simulink library "Byte_Multiplexers_Lib"  (Simulink 8.7)
settings: Solver=ode45  StartTime=0.0  StopTime=10.0  RelTol=1e-3
libraries: commutil2 x34, Bit_Multiplexers_Lib x32, Byte_Multiplexers_Lib x1, Encoders_Lib x1
settings Model: Creator=uzivatel  LastModifiedBy=Jozko Mrkvicka

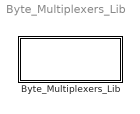
== system Byte_Multiplexers_Lib ==
  Byte_Multiplexers_Lib : Subsystem

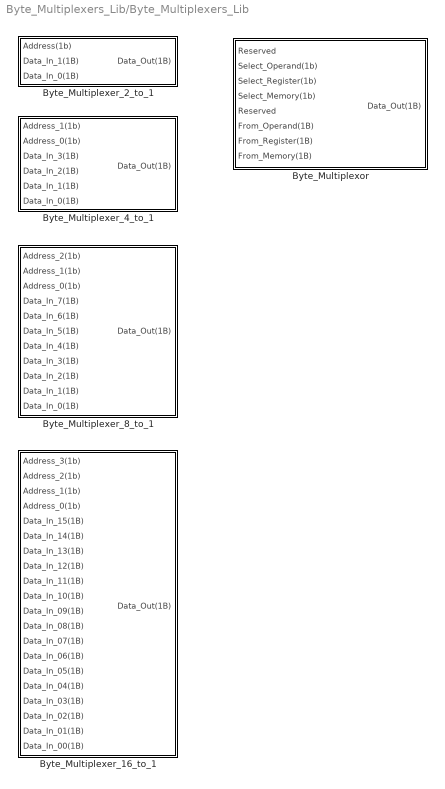
== system Byte_Multiplexers_Lib/Byte_Multiplexers_Lib ==
  Byte_Multiplexer_16_to_1 : Subsystem
  Byte_Multiplexer_2_to_1 : Subsystem
  Byte_Multiplexer_4_to_1 : Subsystem
  Byte_Multiplexer_8_to_1 : Subsystem
  Byte_Multiplexor : Subsystem

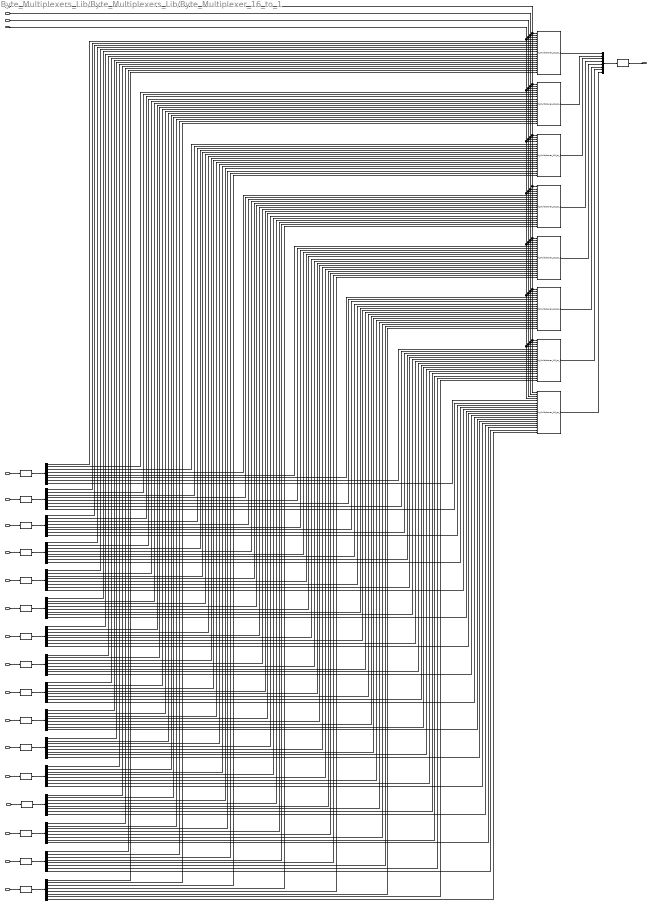
== system Byte_Multiplexers_Lib/Byte_Multiplexers_Lib/Byte_Multiplexer_16_to_1 ==
  Address_3(1b) : Inport
  Address_2(1b) : Inport  Port=2
  Address_1(1b) : Inport  Port=3
  Address_0(1b) : Inport  Port=4
  Data_In_15(1B) : Inport  Port=5
  Data_In_14(1B) : Inport  Port=6
  Data_In_13(1B) : Inport  Port=7
  Data_In_12(1B) : Inport  Port=8
  Data_In_11(1B) : Inport  Port=9
  Data_In_10(1B) : Inport  Port=10
  Data_In_09(1B) : Inport  Port=11
  Data_In_08(1B) : Inport  Port=12
  Data_In_07(1B) : Inport  Port=13
  Data_In_06(1B) : Inport  Port=14
  Data_In_05(1B) : Inport  Port=15
  Data_In_04(1B) : Inport  Port=16
  Data_In_03(1B) : Inport  Port=17
  Data_In_02(1B) : Inport  Port=18
  Data_In_01(1B) : Inport  Port=19
  Data_In_00(1B) : Inport  Port=20
  Bit to Integer Converter1 : commutil2/Bit to Integer Converter  nbits=8  bitOrder=MSB first  signedOutputValues=Unsigned  outDtype=uint8  outDtypeSigned=Inherit via internal rule
  Bit_Multiplexer_16_to_1(Bit_0) : Bit_Multiplexers_Lib/Bit_Multiplexers_Lib/Bit_Multiplexer_16_to_1
  Bit_Multiplexer_16_to_1(Bit_1) : Bit_Multiplexers_Lib/Bit_Multiplexers_Lib/Bit_Multiplexer_16_to_1
  Bit_Multiplexer_16_to_1(Bit_2) : Bit_Multiplexers_Lib/Bit_Multiplexers_Lib/Bit_Multiplexer_16_to_1
  Bit_Multiplexer_16_to_1(Bit_3) : Bit_Multiplexers_Lib/Bit_Multiplexers_Lib/Bit_Multiplexer_16_to_1
  Bit_Multiplexer_16_to_1(Bit_4) : Bit_Multiplexers_Lib/Bit_Multiplexers_Lib/Bit_Multiplexer_16_to_1
  Bit_Multiplexer_16_to_1(Bit_5) : Bit_Multiplexers_Lib/Bit_Multiplexers_Lib/Bit_Multiplexer_16_to_1
  Bit_Multiplexer_16_to_1(Bit_6) : Bit_Multiplexers_Lib/Bit_Multiplexers_Lib/Bit_Multiplexer_16_to_1
  Bit_Multiplexer_16_to_1(Bit_7) : Bit_Multiplexers_Lib/Bit_Multiplexers_Lib/Bit_Multiplexer_16_to_1
  Byte_{0..15} (16 alike) : Demux  Outputs=8
  Integer to Bit Converter{1..16} (16 alike) : commutil2/Integer to Bit Converter  nbits=8  signedInputValues=Unsigned  bitOrder=MSB first  outDtype=boolean
  Mux : Mux  Inputs=8
  Data_Out(1B) : Outport
  wires:
  Integer to Bit Converter7/1 -> Byte_15/1
  Data_In_15(1B)/1 -> Integer to Bit Converter7/1
  Mux/1 -> Bit to Integer Converter1/1
  Bit to Integer Converter1/1 -> Data_Out(1B)/1
  Address_0(1b)/1 -> Bit_Multiplexer_16_to_1(Bit_5)/4, Bit_Multiplexer_16_to_1(Bit_0)/4, Bit_Multiplexer_16_to_1(Bit_1)/4, Bit_Multiplexer_16_to_1(Bit_2)/4, Bit_Multiplexer_16_to_1(Bit_3)/4, Bit_Multiplexer_16_to_1(Bit_4)/4, Bit_Multiplexer_16_to_1(Bit_6)/4, Bit_Multiplexer_16_to_1(Bit_7)/4
  Address_1(1b)/1 -> Bit_Multiplexer_16_to_1(Bit_5)/3, Bit_Multiplexer_16_to_1(Bit_0)/3, Bit_Multiplexer_16_to_1(Bit_1)/3, Bit_Multiplexer_16_to_1(Bit_2)/3, Bit_Multiplexer_16_to_1(Bit_3)/3, Bit_Multiplexer_16_to_1(Bit_4)/3, Bit_Multiplexer_16_to_1(Bit_6)/3, Bit_Multiplexer_16_to_1(Bit_7)/3
  Address_2(1b)/1 -> Bit_Multiplexer_16_to_1(Bit_6)/2, Bit_Multiplexer_16_to_1(Bit_5)/2, Bit_Multiplexer_16_to_1(Bit_4)/2, Bit_Multiplexer_16_to_1(Bit_2)/2, Bit_Multiplexer_16_to_1(Bit_1)/2, Bit_Multiplexer_16_to_1(Bit_0)/2, Bit_Multiplexer_16_to_1(Bit_3)/2, Bit_Multiplexer_16_to_1(Bit_7)/2
  Address_3(1b)/1 -> Bit_Multiplexer_16_to_1(Bit_5)/1, Bit_Multiplexer_16_to_1(Bit_0)/1, Bit_Multiplexer_16_to_1(Bit_1)/1, Bit_Multiplexer_16_to_1(Bit_2)/1, Bit_Multiplexer_16_to_1(Bit_3)/1, Bit_Multiplexer_16_to_1(Bit_4)/1, Bit_Multiplexer_16_to_1(Bit_6)/1, Bit_Multiplexer_16_to_1(Bit_7)/1
  Bit_Multiplexer_16_to_1(Bit_4)/1 -> Mux/4
  Bit_Multiplexer_16_to_1(Bit_5)/1 -> Mux/3
  Bit_Multiplexer_16_to_1(Bit_6)/1 -> Mux/2
  Bit_Multiplexer_16_to_1(Bit_7)/1 -> Mux/1
  Bit_Multiplexer_16_to_1(Bit_3)/1 -> Mux/5
  Bit_Multiplexer_16_to_1(Bit_2)/1 -> Mux/6
  Bit_Multiplexer_16_to_1(Bit_1)/1 -> Mux/7
  Bit_Multiplexer_16_to_1(Bit_0)/1 -> Mux/8
  Integer to Bit Converter1/1 -> Byte_14/1
  Data_In_14(1B)/1 -> Integer to Bit Converter1/1
  Integer to Bit Converter2/1 -> Byte_13/1
  Data_In_13(1B)/1 -> Integer to Bit Converter2/1
  Integer to Bit Converter3/1 -> Byte_12/1
  Data_In_12(1B)/1 -> Integer to Bit Converter3/1
  Integer to Bit Converter4/1 -> Byte_11/1
  Data_In_11(1B)/1 -> Integer to Bit Converter4/1
  Integer to Bit Converter5/1 -> Byte_10/1
  Data_In_10(1B)/1 -> Integer to Bit Converter5/1
  Integer to Bit Converter6/1 -> Byte_9/1
  Data_In_09(1B)/1 -> Integer to Bit Converter6/1
  Integer to Bit Converter8/1 -> Byte_8/1
  Data_In_08(1B)/1 -> Integer to Bit Converter8/1
  Integer to Bit Converter9/1 -> Byte_7/1
  Data_In_07(1B)/1 -> Integer to Bit Converter9/1
  Integer to Bit Converter10/1 -> Byte_6/1
  Data_In_06(1B)/1 -> Integer to Bit Converter10/1
  Integer to Bit Converter11/1 -> Byte_5/1
  Data_In_05(1B)/1 -> Integer to Bit Converter11/1
  Integer to Bit Converter12/1 -> Byte_4/1
  Data_In_04(1B)/1 -> Integer to Bit Converter12/1
  Integer to Bit Converter13/1 -> Byte_3/1
  Data_In_03(1B)/1 -> Integer to Bit Converter13/1
  Integer to Bit Converter14/1 -> Byte_2/1
  Data_In_02(1B)/1 -> Integer to Bit Converter14/1
  Integer to Bit Converter15/1 -> Byte_1/1
  Data_In_01(1B)/1 -> Integer to Bit Converter15/1
  Integer to Bit Converter16/1 -> Byte_0/1
  Data_In_00(1B)/1 -> Integer to Bit Converter16/1
  Byte_15/1 -> Bit_Multiplexer_16_to_1(Bit_7)/5
  Byte_14/1 -> Bit_Multiplexer_16_to_1(Bit_7)/6
  Byte_13/1 -> Bit_Multiplexer_16_to_1(Bit_7)/7
  Byte_12/1 -> Bit_Multiplexer_16_to_1(Bit_7)/8
  Byte_11/1 -> Bit_Multiplexer_16_to_1(Bit_7)/9
  Byte_10/1 -> Bit_Multiplexer_16_to_1(Bit_7)/10
  Byte_9/1 -> Bit_Multiplexer_16_to_1(Bit_7)/11
  Byte_8/1 -> Bit_Multiplexer_16_to_1(Bit_7)/12
  Byte_7/1 -> Bit_Multiplexer_16_to_1(Bit_7)/13
  Byte_6/1 -> Bit_Multiplexer_16_to_1(Bit_7)/14
  Byte_5/1 -> Bit_Multiplexer_16_to_1(Bit_7)/15
  Byte_4/1 -> Bit_Multiplexer_16_to_1(Bit_7)/16
  Byte_3/1 -> Bit_Multiplexer_16_to_1(Bit_7)/17
  Byte_2/1 -> Bit_Multiplexer_16_to_1(Bit_7)/18
  Byte_1/1 -> Bit_Multiplexer_16_to_1(Bit_7)/19
  Byte_0/1 -> Bit_Multiplexer_16_to_1(Bit_7)/20
  Byte_15/2 -> Bit_Multiplexer_16_to_1(Bit_6)/5
  Byte_14/2 -> Bit_Multiplexer_16_to_1(Bit_6)/6
  Byte_13/2 -> Bit_Multiplexer_16_to_1(Bit_6)/7
  Byte_12/2 -> Bit_Multiplexer_16_to_1(Bit_6)/8
  Byte_11/2 -> Bit_Multiplexer_16_to_1(Bit_6)/9
  Byte_10/2 -> Bit_Multiplexer_16_to_1(Bit_6)/10
  Byte_9/2 -> Bit_Multiplexer_16_to_1(Bit_6)/11
  Byte_8/2 -> Bit_Multiplexer_16_to_1(Bit_6)/12
  Byte_7/2 -> Bit_Multiplexer_16_to_1(Bit_6)/13
  Byte_6/2 -> Bit_Multiplexer_16_to_1(Bit_6)/14
  Byte_5/2 -> Bit_Multiplexer_16_to_1(Bit_6)/15
  Byte_4/2 -> Bit_Multiplexer_16_to_1(Bit_6)/16
  Byte_3/2 -> Bit_Multiplexer_16_to_1(Bit_6)/17
  Byte_2/2 -> Bit_Multiplexer_16_to_1(Bit_6)/18
  Byte_1/2 -> Bit_Multiplexer_16_to_1(Bit_6)/19
  Byte_0/2 -> Bit_Multiplexer_16_to_1(Bit_6)/20
  Byte_15/3 -> Bit_Multiplexer_16_to_1(Bit_5)/5
  Byte_14/3 -> Bit_Multiplexer_16_to_1(Bit_5)/6
  Byte_13/3 -> Bit_Multiplexer_16_to_1(Bit_5)/7
  Byte_12/3 -> Bit_Multiplexer_16_to_1(Bit_5)/8
  Byte_11/3 -> Bit_Multiplexer_16_to_1(Bit_5)/9
  Byte_10/3 -> Bit_Multiplexer_16_to_1(Bit_5)/10
  Byte_9/3 -> Bit_Multiplexer_16_to_1(Bit_5)/11
  Byte_8/3 -> Bit_Multiplexer_16_to_1(Bit_5)/12
  Byte_7/3 -> Bit_Multiplexer_16_to_1(Bit_5)/13
  Byte_6/3 -> Bit_Multiplexer_16_to_1(Bit_5)/14
  Byte_5/3 -> Bit_Multiplexer_16_to_1(Bit_5)/15
  Byte_4/3 -> Bit_Multiplexer_16_to_1(Bit_5)/16
  Byte_3/3 -> Bit_Multiplexer_16_to_1(Bit_5)/17
  Byte_2/3 -> Bit_Multiplexer_16_to_1(Bit_5)/18
  Byte_1/3 -> Bit_Multiplexer_16_to_1(Bit_5)/19
  Byte_0/3 -> Bit_Multiplexer_16_to_1(Bit_5)/20
  Byte_15/4 -> Bit_Multiplexer_16_to_1(Bit_4)/5
  Byte_14/4 -> Bit_Multiplexer_16_to_1(Bit_4)/6
  Byte_13/4 -> Bit_Multiplexer_16_to_1(Bit_4)/7
  Byte_12/4 -> Bit_Multiplexer_16_to_1(Bit_4)/8
  Byte_11/4 -> Bit_Multiplexer_16_to_1(Bit_4)/9
  Byte_10/4 -> Bit_Multiplexer_16_to_1(Bit_4)/10
  Byte_9/4 -> Bit_Multiplexer_16_to_1(Bit_4)/11
  Byte_8/4 -> Bit_Multiplexer_16_to_1(Bit_4)/12
  Byte_7/4 -> Bit_Multiplexer_16_to_1(Bit_4)/13
  Byte_6/4 -> Bit_Multiplexer_16_to_1(Bit_4)/14
  Byte_5/4 -> Bit_Multiplexer_16_to_1(Bit_4)/15
  Byte_4/4 -> Bit_Multiplexer_16_to_1(Bit_4)/16
  Byte_3/4 -> Bit_Multiplexer_16_to_1(Bit_4)/17
  Byte_2/4 -> Bit_Multiplexer_16_to_1(Bit_4)/18
  Byte_1/4 -> Bit_Multiplexer_16_to_1(Bit_4)/19
  Byte_0/4 -> Bit_Multiplexer_16_to_1(Bit_4)/20
  Byte_15/5 -> Bit_Multiplexer_16_to_1(Bit_3)/5
  Byte_14/5 -> Bit_Multiplexer_16_to_1(Bit_3)/6
  Byte_13/5 -> Bit_Multiplexer_16_to_1(Bit_3)/7
  Byte_12/5 -> Bit_Multiplexer_16_to_1(Bit_3)/8
  Byte_11/5 -> Bit_Multiplexer_16_to_1(Bit_3)/9
  Byte_10/5 -> Bit_Multiplexer_16_to_1(Bit_3)/10
  Byte_9/5 -> Bit_Multiplexer_16_to_1(Bit_3)/11
  Byte_8/5 -> Bit_Multiplexer_16_to_1(Bit_3)/12
  Byte_7/5 -> Bit_Multiplexer_16_to_1(Bit_3)/13
  Byte_6/5 -> Bit_Multiplexer_16_to_1(Bit_3)/14
  Byte_5/5 -> Bit_Multiplexer_16_to_1(Bit_3)/15
  Byte_4/5 -> Bit_Multiplexer_16_to_1(Bit_3)/16
  Byte_3/5 -> Bit_Multiplexer_16_to_1(Bit_3)/17
  Byte_2/5 -> Bit_Multiplexer_16_to_1(Bit_3)/18
  Byte_1/5 -> Bit_Multiplexer_16_to_1(Bit_3)/19
  Byte_0/5 -> Bit_Multiplexer_16_to_1(Bit_3)/20
  Byte_15/6 -> Bit_Multiplexer_16_to_1(Bit_2)/5
  Byte_14/6 -> Bit_Multiplexer_16_to_1(Bit_2)/6
  Byte_13/6 -> Bit_Multiplexer_16_to_1(Bit_2)/7
  Byte_12/6 -> Bit_Multiplexer_16_to_1(Bit_2)/8
  Byte_11/6 -> Bit_Multiplexer_16_to_1(Bit_2)/9
  Byte_10/6 -> Bit_Multiplexer_16_to_1(Bit_2)/10
  Byte_9/6 -> Bit_Multiplexer_16_to_1(Bit_2)/11
  Byte_8/6 -> Bit_Multiplexer_16_to_1(Bit_2)/12
  Byte_7/6 -> Bit_Multiplexer_16_to_1(Bit_2)/13
  Byte_6/6 -> Bit_Multiplexer_16_to_1(Bit_2)/14
  Byte_5/6 -> Bit_Multiplexer_16_to_1(Bit_2)/15
  Byte_4/6 -> Bit_Multiplexer_16_to_1(Bit_2)/16
  Byte_3/6 -> Bit_Multiplexer_16_to_1(Bit_2)/17
  Byte_2/6 -> Bit_Multiplexer_16_to_1(Bit_2)/18
  Byte_1/6 -> Bit_Multiplexer_16_to_1(Bit_2)/19
  Byte_0/6 -> Bit_Multiplexer_16_to_1(Bit_2)/20
  Byte_15/7 -> Bit_Multiplexer_16_to_1(Bit_1)/5
  Byte_14/7 -> Bit_Multiplexer_16_to_1(Bit_1)/6
  Byte_13/7 -> Bit_Multiplexer_16_to_1(Bit_1)/7
  Byte_12/7 -> Bit_Multiplexer_16_to_1(Bit_1)/8
  Byte_11/7 -> Bit_Multiplexer_16_to_1(Bit_1)/9
  Byte_10/7 -> Bit_Multiplexer_16_to_1(Bit_1)/10
  Byte_9/7 -> Bit_Multiplexer_16_to_1(Bit_1)/11
  Byte_8/7 -> Bit_Multiplexer_16_to_1(Bit_1)/12
  Byte_7/7 -> Bit_Multiplexer_16_to_1(Bit_1)/13
  Byte_6/7 -> Bit_Multiplexer_16_to_1(Bit_1)/14
  Byte_5/7 -> Bit_Multiplexer_16_to_1(Bit_1)/15
  Byte_4/7 -> Bit_Multiplexer_16_to_1(Bit_1)/16
  Byte_3/7 -> Bit_Multiplexer_16_to_1(Bit_1)/17
  Byte_2/7 -> Bit_Multiplexer_16_to_1(Bit_1)/18
  Byte_1/7 -> Bit_Multiplexer_16_to_1(Bit_1)/19
  Byte_0/7 -> Bit_Multiplexer_16_to_1(Bit_1)/20
  Byte_15/8 -> Bit_Multiplexer_16_to_1(Bit_0)/5
  Byte_14/8 -> Bit_Multiplexer_16_to_1(Bit_0)/6
  Byte_13/8 -> Bit_Multiplexer_16_to_1(Bit_0)/7
  Byte_12/8 -> Bit_Multiplexer_16_to_1(Bit_0)/8
  Byte_11/8 -> Bit_Multiplexer_16_to_1(Bit_0)/9
  Byte_10/8 -> Bit_Multiplexer_16_to_1(Bit_0)/10
  Byte_9/8 -> Bit_Multiplexer_16_to_1(Bit_0)/11
  Byte_8/8 -> Bit_Multiplexer_16_to_1(Bit_0)/12
  Byte_7/8 -> Bit_Multiplexer_16_to_1(Bit_0)/13
  Byte_6/8 -> Bit_Multiplexer_16_to_1(Bit_0)/14
  Byte_5/8 -> Bit_Multiplexer_16_to_1(Bit_0)/15
  Byte_4/8 -> Bit_Multiplexer_16_to_1(Bit_0)/16
  Byte_3/8 -> Bit_Multiplexer_16_to_1(Bit_0)/17
  Byte_2/8 -> Bit_Multiplexer_16_to_1(Bit_0)/18
  Byte_1/8 -> Bit_Multiplexer_16_to_1(Bit_0)/19
  Byte_0/8 -> Bit_Multiplexer_16_to_1(Bit_0)/20

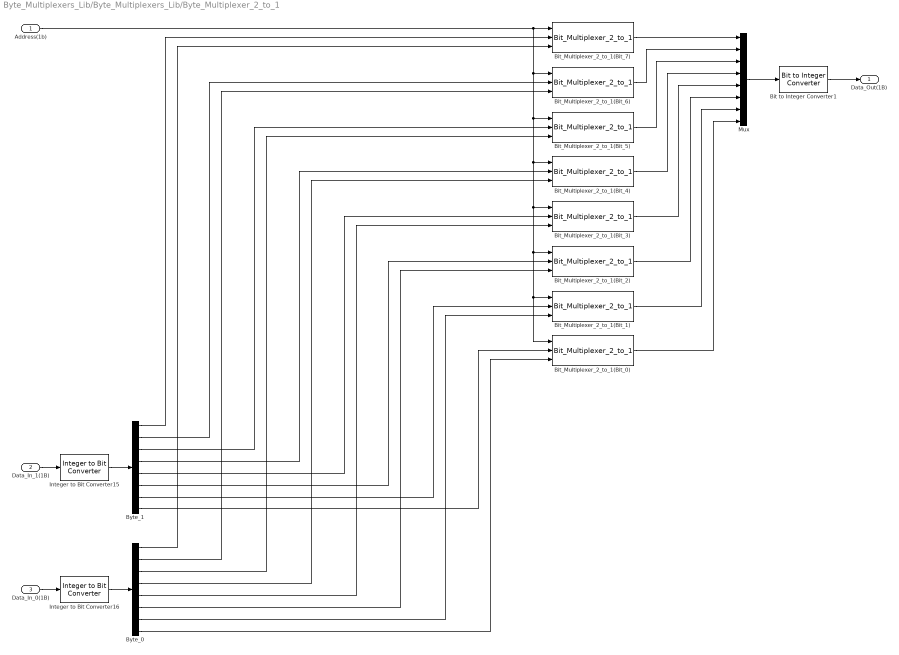
== system Byte_Multiplexers_Lib/Byte_Multiplexers_Lib/Byte_Multiplexer_2_to_1 ==
  Address(1b) : Inport
  Data_In_1(1B) : Inport  Port=2
  Data_In_0(1B) : Inport  Port=3
  Bit to Integer Converter1 : commutil2/Bit to Integer Converter  nbits=8  bitOrder=MSB first  signedOutputValues=Unsigned  outDtype=uint8  outDtypeSigned=Inherit via internal rule
  Bit_Multiplexer_2_to_1(Bit_0) : Bit_Multiplexers_Lib/Bit_Multiplexers_Lib/Bit_Multiplexer_2_to_1
  Bit_Multiplexer_2_to_1(Bit_1) : Bit_Multiplexers_Lib/Bit_Multiplexers_Lib/Bit_Multiplexer_2_to_1
  Bit_Multiplexer_2_to_1(Bit_2) : Bit_Multiplexers_Lib/Bit_Multiplexers_Lib/Bit_Multiplexer_2_to_1
  Bit_Multiplexer_2_to_1(Bit_3) : Bit_Multiplexers_Lib/Bit_Multiplexers_Lib/Bit_Multiplexer_2_to_1
  Bit_Multiplexer_2_to_1(Bit_4) : Bit_Multiplexers_Lib/Bit_Multiplexers_Lib/Bit_Multiplexer_2_to_1
  Bit_Multiplexer_2_to_1(Bit_5) : Bit_Multiplexers_Lib/Bit_Multiplexers_Lib/Bit_Multiplexer_2_to_1
  Bit_Multiplexer_2_to_1(Bit_6) : Bit_Multiplexers_Lib/Bit_Multiplexers_Lib/Bit_Multiplexer_2_to_1
  Bit_Multiplexer_2_to_1(Bit_7) : Bit_Multiplexers_Lib/Bit_Multiplexers_Lib/Bit_Multiplexer_2_to_1
  Byte_0 : Demux  Outputs=8
  Byte_1 : Demux  Outputs=8
  Integer to Bit Converter15 : commutil2/Integer to Bit Converter  nbits=8  signedInputValues=Unsigned  bitOrder=MSB first  outDtype=boolean
  Integer to Bit Converter16 : commutil2/Integer to Bit Converter  nbits=8  signedInputValues=Unsigned  bitOrder=MSB first  outDtype=boolean
  Mux : Mux  Inputs=8
  Data_Out(1B) : Outport
  wires:
  Mux/1 -> Bit to Integer Converter1/1
  Bit to Integer Converter1/1 -> Data_Out(1B)/1
  Address(1b)/1 -> Bit_Multiplexer_2_to_1(Bit_7)/1, Bit_Multiplexer_2_to_1(Bit_0)/1, Bit_Multiplexer_2_to_1(Bit_1)/1, Bit_Multiplexer_2_to_1(Bit_2)/1, Bit_Multiplexer_2_to_1(Bit_3)/1, Bit_Multiplexer_2_to_1(Bit_4)/1, Bit_Multiplexer_2_to_1(Bit_5)/1, Bit_Multiplexer_2_to_1(Bit_6)/1
  Bit_Multiplexer_2_to_1(Bit_4)/1 -> Mux/4
  Bit_Multiplexer_2_to_1(Bit_5)/1 -> Mux/3
  Bit_Multiplexer_2_to_1(Bit_6)/1 -> Mux/2
  Bit_Multiplexer_2_to_1(Bit_7)/1 -> Mux/1
  Bit_Multiplexer_2_to_1(Bit_3)/1 -> Mux/5
  Bit_Multiplexer_2_to_1(Bit_2)/1 -> Mux/6
  Bit_Multiplexer_2_to_1(Bit_1)/1 -> Mux/7
  Bit_Multiplexer_2_to_1(Bit_0)/1 -> Mux/8
  Integer to Bit Converter15/1 -> Byte_1/1
  Data_In_1(1B)/1 -> Integer to Bit Converter15/1
  Integer to Bit Converter16/1 -> Byte_0/1
  Data_In_0(1B)/1 -> Integer to Bit Converter16/1
  Byte_1/8 -> Bit_Multiplexer_2_to_1(Bit_0)/2
  Byte_0/8 -> Bit_Multiplexer_2_to_1(Bit_0)/3
  Byte_1/7 -> Bit_Multiplexer_2_to_1(Bit_1)/2
  Byte_0/7 -> Bit_Multiplexer_2_to_1(Bit_1)/3
  Byte_1/6 -> Bit_Multiplexer_2_to_1(Bit_2)/2
  Byte_0/6 -> Bit_Multiplexer_2_to_1(Bit_2)/3
  Byte_0/5 -> Bit_Multiplexer_2_to_1(Bit_3)/3
  Byte_1/5 -> Bit_Multiplexer_2_to_1(Bit_3)/2
  Byte_0/4 -> Bit_Multiplexer_2_to_1(Bit_4)/3
  Byte_1/4 -> Bit_Multiplexer_2_to_1(Bit_4)/2
  Byte_1/3 -> Bit_Multiplexer_2_to_1(Bit_5)/2
  Byte_0/3 -> Bit_Multiplexer_2_to_1(Bit_5)/3
  Byte_1/2 -> Bit_Multiplexer_2_to_1(Bit_6)/2
  Byte_0/2 -> Bit_Multiplexer_2_to_1(Bit_6)/3
  Byte_0/1 -> Bit_Multiplexer_2_to_1(Bit_7)/3
  Byte_1/1 -> Bit_Multiplexer_2_to_1(Bit_7)/2

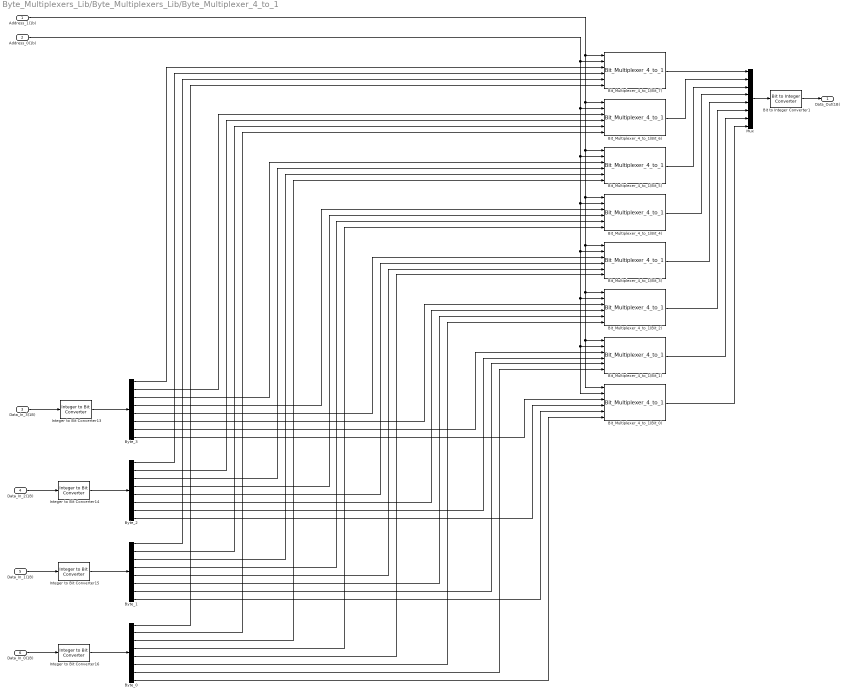
== system Byte_Multiplexers_Lib/Byte_Multiplexers_Lib/Byte_Multiplexer_4_to_1 ==
  Address_1(1b) : Inport
  Address_0(1b) : Inport  Port=2
  Data_In_3(1B) : Inport  Port=3
  Data_In_2(1B) : Inport  Port=4
  Data_In_1(1B) : Inport  Port=5
  Data_In_0(1B) : Inport  Port=6
  Bit to Integer Converter1 : commutil2/Bit to Integer Converter  nbits=8  bitOrder=MSB first  signedOutputValues=Unsigned  outDtype=uint8  outDtypeSigned=Inherit via internal rule
  Bit_Multiplexer_4_to_1(Bit_0) : Bit_Multiplexers_Lib/Bit_Multiplexers_Lib/Bit_Multiplexer_4_to_1
  Bit_Multiplexer_4_to_1(Bit_1) : Bit_Multiplexers_Lib/Bit_Multiplexers_Lib/Bit_Multiplexer_4_to_1
  Bit_Multiplexer_4_to_1(Bit_2) : Bit_Multiplexers_Lib/Bit_Multiplexers_Lib/Bit_Multiplexer_4_to_1
  Bit_Multiplexer_4_to_1(Bit_3) : Bit_Multiplexers_Lib/Bit_Multiplexers_Lib/Bit_Multiplexer_4_to_1
  Bit_Multiplexer_4_to_1(Bit_4) : Bit_Multiplexers_Lib/Bit_Multiplexers_Lib/Bit_Multiplexer_4_to_1
  Bit_Multiplexer_4_to_1(Bit_5) : Bit_Multiplexers_Lib/Bit_Multiplexers_Lib/Bit_Multiplexer_4_to_1
  Bit_Multiplexer_4_to_1(Bit_6) : Bit_Multiplexers_Lib/Bit_Multiplexers_Lib/Bit_Multiplexer_4_to_1
  Bit_Multiplexer_4_to_1(Bit_7) : Bit_Multiplexers_Lib/Bit_Multiplexers_Lib/Bit_Multiplexer_4_to_1
  Byte_{0..3} (4 alike) : Demux  Outputs=8
  Integer to Bit Converter{13..16} (4 alike) : commutil2/Integer to Bit Converter  nbits=8  signedInputValues=Unsigned  bitOrder=MSB first  outDtype=boolean
  Mux : Mux  Inputs=8
  Data_Out(1B) : Outport
  wires:
  Mux/1 -> Bit to Integer Converter1/1
  Bit to Integer Converter1/1 -> Data_Out(1B)/1
  Address_0(1b)/1 -> Bit_Multiplexer_4_to_1(Bit_0)/2, Bit_Multiplexer_4_to_1(Bit_1)/2, Bit_Multiplexer_4_to_1(Bit_2)/2, Bit_Multiplexer_4_to_1(Bit_3)/2, Bit_Multiplexer_4_to_1(Bit_4)/2, Bit_Multiplexer_4_to_1(Bit_5)/2, Bit_Multiplexer_4_to_1(Bit_6)/2, Bit_Multiplexer_4_to_1(Bit_7)/2
  Address_1(1b)/1 -> Bit_Multiplexer_4_to_1(Bit_7)/1, Bit_Multiplexer_4_to_1(Bit_0)/1, Bit_Multiplexer_4_to_1(Bit_1)/1, Bit_Multiplexer_4_to_1(Bit_2)/1, Bit_Multiplexer_4_to_1(Bit_3)/1, Bit_Multiplexer_4_to_1(Bit_4)/1, Bit_Multiplexer_4_to_1(Bit_5)/1, Bit_Multiplexer_4_to_1(Bit_6)/1
  Bit_Multiplexer_4_to_1(Bit_4)/1 -> Mux/4
  Bit_Multiplexer_4_to_1(Bit_5)/1 -> Mux/3
  Bit_Multiplexer_4_to_1(Bit_6)/1 -> Mux/2
  Bit_Multiplexer_4_to_1(Bit_7)/1 -> Mux/1
  Bit_Multiplexer_4_to_1(Bit_3)/1 -> Mux/5
  Bit_Multiplexer_4_to_1(Bit_2)/1 -> Mux/6
  Bit_Multiplexer_4_to_1(Bit_1)/1 -> Mux/7
  Bit_Multiplexer_4_to_1(Bit_0)/1 -> Mux/8
  Integer to Bit Converter13/1 -> Byte_3/1
  Data_In_3(1B)/1 -> Integer to Bit Converter13/1
  Integer to Bit Converter14/1 -> Byte_2/1
  Data_In_2(1B)/1 -> Integer to Bit Converter14/1
  Integer to Bit Converter15/1 -> Byte_1/1
  Data_In_1(1B)/1 -> Integer to Bit Converter15/1
  Integer to Bit Converter16/1 -> Byte_0/1
  Data_In_0(1B)/1 -> Integer to Bit Converter16/1
  Byte_3/8 -> Bit_Multiplexer_4_to_1(Bit_0)/3
  Byte_2/8 -> Bit_Multiplexer_4_to_1(Bit_0)/4
  Byte_1/8 -> Bit_Multiplexer_4_to_1(Bit_0)/5
  Byte_0/8 -> Bit_Multiplexer_4_to_1(Bit_0)/6
  Byte_3/7 -> Bit_Multiplexer_4_to_1(Bit_1)/3
  Byte_2/7 -> Bit_Multiplexer_4_to_1(Bit_1)/4
  Byte_1/7 -> Bit_Multiplexer_4_to_1(Bit_1)/5
  Byte_0/7 -> Bit_Multiplexer_4_to_1(Bit_1)/6
  Byte_3/6 -> Bit_Multiplexer_4_to_1(Bit_2)/3
  Byte_2/6 -> Bit_Multiplexer_4_to_1(Bit_2)/4
  Byte_1/6 -> Bit_Multiplexer_4_to_1(Bit_2)/5
  Byte_0/6 -> Bit_Multiplexer_4_to_1(Bit_2)/6
  Byte_3/5 -> Bit_Multiplexer_4_to_1(Bit_3)/3
  Byte_2/5 -> Bit_Multiplexer_4_to_1(Bit_3)/4
  Byte_1/5 -> Bit_Multiplexer_4_to_1(Bit_3)/5
  Byte_0/5 -> Bit_Multiplexer_4_to_1(Bit_3)/6
  Byte_3/4 -> Bit_Multiplexer_4_to_1(Bit_4)/3
  Byte_2/4 -> Bit_Multiplexer_4_to_1(Bit_4)/4
  Byte_1/4 -> Bit_Multiplexer_4_to_1(Bit_4)/5
  Byte_0/4 -> Bit_Multiplexer_4_to_1(Bit_4)/6
  Byte_3/3 -> Bit_Multiplexer_4_to_1(Bit_5)/3
  Byte_2/3 -> Bit_Multiplexer_4_to_1(Bit_5)/4
  Byte_1/3 -> Bit_Multiplexer_4_to_1(Bit_5)/5
  Byte_0/3 -> Bit_Multiplexer_4_to_1(Bit_5)/6
  Byte_3/2 -> Bit_Multiplexer_4_to_1(Bit_6)/3
  Byte_2/2 -> Bit_Multiplexer_4_to_1(Bit_6)/4
  Byte_1/2 -> Bit_Multiplexer_4_to_1(Bit_6)/5
  Byte_0/2 -> Bit_Multiplexer_4_to_1(Bit_6)/6
  Byte_3/1 -> Bit_Multiplexer_4_to_1(Bit_7)/3
  Byte_2/1 -> Bit_Multiplexer_4_to_1(Bit_7)/4
  Byte_1/1 -> Bit_Multiplexer_4_to_1(Bit_7)/5
  Byte_0/1 -> Bit_Multiplexer_4_to_1(Bit_7)/6

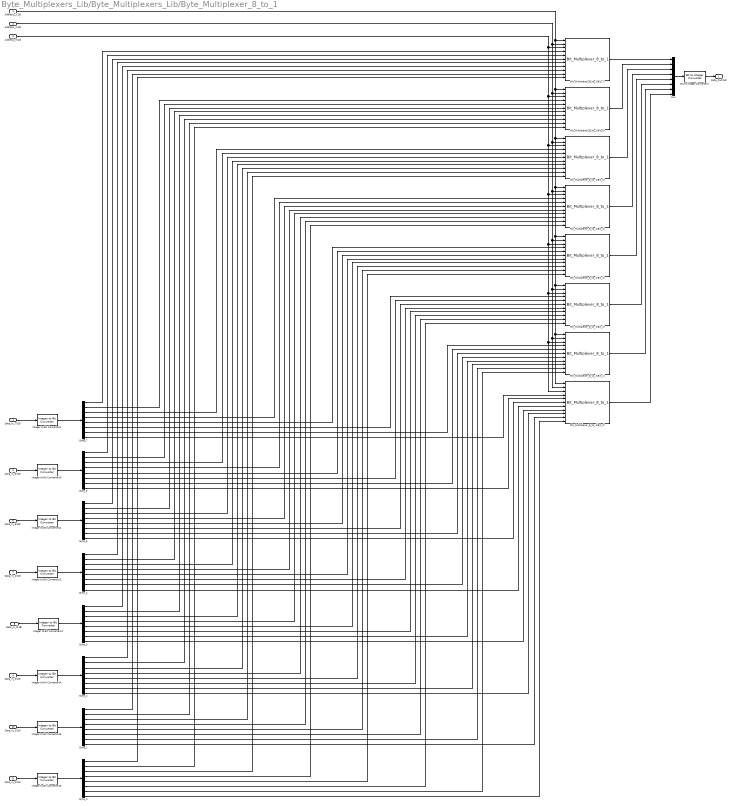
== system Byte_Multiplexers_Lib/Byte_Multiplexers_Lib/Byte_Multiplexer_8_to_1 ==
  Address_2(1b) : Inport
  Address_1(1b) : Inport  Port=2
  Address_0(1b) : Inport  Port=3
  Data_In_7(1B) : Inport  Port=4
  Data_In_6(1B) : Inport  Port=5
  Data_In_5(1B) : Inport  Port=6
  Data_In_4(1B) : Inport  Port=7
  Data_In_3(1B) : Inport  Port=8
  Data_In_2(1B) : Inport  Port=9
  Data_In_1(1B) : Inport  Port=10
  Data_In_0(1B) : Inport  Port=11
  Bit to Integer Converter1 : commutil2/Bit to Integer Converter  nbits=8  bitOrder=MSB first  signedOutputValues=Unsigned  outDtype=uint8  outDtypeSigned=Inherit via internal rule
  Bit_Multiplexer_8_to_1(Bit_0) : Bit_Multiplexers_Lib/Bit_Multiplexers_Lib/Bit_Multiplexer_8_to_1
  Bit_Multiplexer_8_to_1(Bit_1) : Bit_Multiplexers_Lib/Bit_Multiplexers_Lib/Bit_Multiplexer_8_to_1
  Bit_Multiplexer_8_to_1(Bit_2) : Bit_Multiplexers_Lib/Bit_Multiplexers_Lib/Bit_Multiplexer_8_to_1
  Bit_Multiplexer_8_to_1(Bit_3) : Bit_Multiplexers_Lib/Bit_Multiplexers_Lib/Bit_Multiplexer_8_to_1
  Bit_Multiplexer_8_to_1(Bit_4) : Bit_Multiplexers_Lib/Bit_Multiplexers_Lib/Bit_Multiplexer_8_to_1
  Bit_Multiplexer_8_to_1(Bit_5) : Bit_Multiplexers_Lib/Bit_Multiplexers_Lib/Bit_Multiplexer_8_to_1
  Bit_Multiplexer_8_to_1(Bit_6) : Bit_Multiplexers_Lib/Bit_Multiplexers_Lib/Bit_Multiplexer_8_to_1
  Bit_Multiplexer_8_to_1(Bit_7) : Bit_Multiplexers_Lib/Bit_Multiplexers_Lib/Bit_Multiplexer_8_to_1
  Byte_{0..7} (8 alike) : Demux  Outputs=8
  Integer to Bit Converter{9..16} (8 alike) : commutil2/Integer to Bit Converter  nbits=8  signedInputValues=Unsigned  bitOrder=MSB first  outDtype=boolean
  Mux : Mux  Inputs=8
  Data_Out(1B) : Outport
  wires:
  Mux/1 -> Bit to Integer Converter1/1
  Bit to Integer Converter1/1 -> Data_Out(1B)/1
  Address_0(1b)/1 -> Bit_Multiplexer_8_to_1(Bit_0)/3, Bit_Multiplexer_8_to_1(Bit_1)/3, Bit_Multiplexer_8_to_1(Bit_2)/3, Bit_Multiplexer_8_to_1(Bit_3)/3, Bit_Multiplexer_8_to_1(Bit_4)/3, Bit_Multiplexer_8_to_1(Bit_5)/3, Bit_Multiplexer_8_to_1(Bit_6)/3, Bit_Multiplexer_8_to_1(Bit_7)/3
  Address_1(1b)/1 -> Bit_Multiplexer_8_to_1(Bit_5)/2, Bit_Multiplexer_8_to_1(Bit_0)/2, Bit_Multiplexer_8_to_1(Bit_1)/2, Bit_Multiplexer_8_to_1(Bit_2)/2, Bit_Multiplexer_8_to_1(Bit_3)/2, Bit_Multiplexer_8_to_1(Bit_4)/2, Bit_Multiplexer_8_to_1(Bit_6)/2, Bit_Multiplexer_8_to_1(Bit_7)/2
  Address_2(1b)/1 -> Bit_Multiplexer_8_to_1(Bit_0)/1, Bit_Multiplexer_8_to_1(Bit_1)/1, Bit_Multiplexer_8_to_1(Bit_2)/1, Bit_Multiplexer_8_to_1(Bit_3)/1, Bit_Multiplexer_8_to_1(Bit_4)/1, Bit_Multiplexer_8_to_1(Bit_5)/1, Bit_Multiplexer_8_to_1(Bit_6)/1, Bit_Multiplexer_8_to_1(Bit_7)/1
  Bit_Multiplexer_8_to_1(Bit_4)/1 -> Mux/4
  Bit_Multiplexer_8_to_1(Bit_5)/1 -> Mux/3
  Bit_Multiplexer_8_to_1(Bit_6)/1 -> Mux/2
  Bit_Multiplexer_8_to_1(Bit_7)/1 -> Mux/1
  Bit_Multiplexer_8_to_1(Bit_3)/1 -> Mux/5
  Bit_Multiplexer_8_to_1(Bit_2)/1 -> Mux/6
  Bit_Multiplexer_8_to_1(Bit_1)/1 -> Mux/7
  Bit_Multiplexer_8_to_1(Bit_0)/1 -> Mux/8
  Integer to Bit Converter9/1 -> Byte_7/1
  Data_In_7(1B)/1 -> Integer to Bit Converter9/1
  Integer to Bit Converter10/1 -> Byte_6/1
  Data_In_6(1B)/1 -> Integer to Bit Converter10/1
  Integer to Bit Converter11/1 -> Byte_5/1
  Data_In_5(1B)/1 -> Integer to Bit Converter11/1
  Integer to Bit Converter12/1 -> Byte_4/1
  Data_In_4(1B)/1 -> Integer to Bit Converter12/1
  Integer to Bit Converter13/1 -> Byte_3/1
  Data_In_3(1B)/1 -> Integer to Bit Converter13/1
  Integer to Bit Converter14/1 -> Byte_2/1
  Data_In_2(1B)/1 -> Integer to Bit Converter14/1
  Integer to Bit Converter15/1 -> Byte_1/1
  Data_In_1(1B)/1 -> Integer to Bit Converter15/1
  Integer to Bit Converter16/1 -> Byte_0/1
  Data_In_0(1B)/1 -> Integer to Bit Converter16/1
  Byte_7/1 -> Bit_Multiplexer_8_to_1(Bit_7)/4
  Byte_6/1 -> Bit_Multiplexer_8_to_1(Bit_7)/5
  Byte_5/1 -> Bit_Multiplexer_8_to_1(Bit_7)/6
  Byte_4/1 -> Bit_Multiplexer_8_to_1(Bit_7)/7
  Byte_3/1 -> Bit_Multiplexer_8_to_1(Bit_7)/8
  Byte_2/1 -> Bit_Multiplexer_8_to_1(Bit_7)/9
  Byte_1/1 -> Bit_Multiplexer_8_to_1(Bit_7)/10
  Byte_0/1 -> Bit_Multiplexer_8_to_1(Bit_7)/11
  Byte_7/2 -> Bit_Multiplexer_8_to_1(Bit_6)/4
  Byte_6/2 -> Bit_Multiplexer_8_to_1(Bit_6)/5
  Byte_5/2 -> Bit_Multiplexer_8_to_1(Bit_6)/6
  Byte_4/2 -> Bit_Multiplexer_8_to_1(Bit_6)/7
  Byte_3/2 -> Bit_Multiplexer_8_to_1(Bit_6)/8
  Byte_2/2 -> Bit_Multiplexer_8_to_1(Bit_6)/9
  Byte_1/2 -> Bit_Multiplexer_8_to_1(Bit_6)/10
  Byte_0/2 -> Bit_Multiplexer_8_to_1(Bit_6)/11
  Byte_7/3 -> Bit_Multiplexer_8_to_1(Bit_5)/4
  Byte_6/3 -> Bit_Multiplexer_8_to_1(Bit_5)/5
  Byte_5/3 -> Bit_Multiplexer_8_to_1(Bit_5)/6
  Byte_4/3 -> Bit_Multiplexer_8_to_1(Bit_5)/7
  Byte_3/3 -> Bit_Multiplexer_8_to_1(Bit_5)/8
  Byte_2/3 -> Bit_Multiplexer_8_to_1(Bit_5)/9
  Byte_1/3 -> Bit_Multiplexer_8_to_1(Bit_5)/10
  Byte_0/3 -> Bit_Multiplexer_8_to_1(Bit_5)/11
  Byte_7/4 -> Bit_Multiplexer_8_to_1(Bit_4)/4
  Byte_6/4 -> Bit_Multiplexer_8_to_1(Bit_4)/5
  Byte_5/4 -> Bit_Multiplexer_8_to_1(Bit_4)/6
  Byte_4/4 -> Bit_Multiplexer_8_to_1(Bit_4)/7
  Byte_3/4 -> Bit_Multiplexer_8_to_1(Bit_4)/8
  Byte_2/4 -> Bit_Multiplexer_8_to_1(Bit_4)/9
  Byte_1/4 -> Bit_Multiplexer_8_to_1(Bit_4)/10
  Byte_0/4 -> Bit_Multiplexer_8_to_1(Bit_4)/11
  Byte_7/5 -> Bit_Multiplexer_8_to_1(Bit_3)/4
  Byte_6/5 -> Bit_Multiplexer_8_to_1(Bit_3)/5
  Byte_5/5 -> Bit_Multiplexer_8_to_1(Bit_3)/6
  Byte_4/5 -> Bit_Multiplexer_8_to_1(Bit_3)/7
  Byte_3/5 -> Bit_Multiplexer_8_to_1(Bit_3)/8
  Byte_2/5 -> Bit_Multiplexer_8_to_1(Bit_3)/9
  Byte_1/5 -> Bit_Multiplexer_8_to_1(Bit_3)/10
  Byte_0/5 -> Bit_Multiplexer_8_to_1(Bit_3)/11
  Byte_7/6 -> Bit_Multiplexer_8_to_1(Bit_2)/4
  Byte_6/6 -> Bit_Multiplexer_8_to_1(Bit_2)/5
  Byte_5/6 -> Bit_Multiplexer_8_to_1(Bit_2)/6
  Byte_4/6 -> Bit_Multiplexer_8_to_1(Bit_2)/7
  Byte_3/6 -> Bit_Multiplexer_8_to_1(Bit_2)/8
  Byte_2/6 -> Bit_Multiplexer_8_to_1(Bit_2)/9
  Byte_1/6 -> Bit_Multiplexer_8_to_1(Bit_2)/10
  Byte_0/6 -> Bit_Multiplexer_8_to_1(Bit_2)/11
  Byte_7/7 -> Bit_Multiplexer_8_to_1(Bit_1)/4
  Byte_6/7 -> Bit_Multiplexer_8_to_1(Bit_1)/5
  Byte_5/7 -> Bit_Multiplexer_8_to_1(Bit_1)/6
  Byte_4/7 -> Bit_Multiplexer_8_to_1(Bit_1)/7
  Byte_3/7 -> Bit_Multiplexer_8_to_1(Bit_1)/8
  Byte_2/7 -> Bit_Multiplexer_8_to_1(Bit_1)/9
  Byte_1/7 -> Bit_Multiplexer_8_to_1(Bit_1)/10
  Byte_0/7 -> Bit_Multiplexer_8_to_1(Bit_1)/11
  Byte_7/8 -> Bit_Multiplexer_8_to_1(Bit_0)/4
  Byte_6/8 -> Bit_Multiplexer_8_to_1(Bit_0)/5
  Byte_5/8 -> Bit_Multiplexer_8_to_1(Bit_0)/6
  Byte_4/8 -> Bit_Multiplexer_8_to_1(Bit_0)/7
  Byte_3/8 -> Bit_Multiplexer_8_to_1(Bit_0)/8
  Byte_2/8 -> Bit_Multiplexer_8_to_1(Bit_0)/9
  Byte_1/8 -> Bit_Multiplexer_8_to_1(Bit_0)/10
  Byte_0/8 -> Bit_Multiplexer_8_to_1(Bit_0)/11

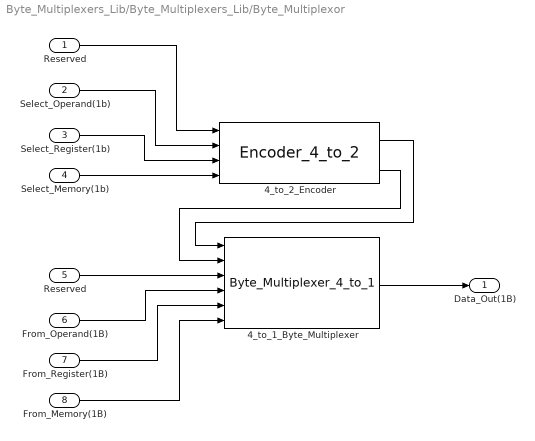
== system Byte_Multiplexers_Lib/Byte_Multiplexers_Lib/Byte_Multiplexor ==
  Reserved : Inport
  Select_Operand(1b) : Inport  Port=2
  Select_Register(1b) : Inport  Port=3
  "Select_Memory(1b) " : Inport  Port=4
  "Reserved " : Inport  Port=5
  From_Operand(1B) : Inport  Port=6
  From_Register(1B) : Inport  Port=7
  From_Memory(1B) : Inport  Port=8
  4_to_1_Byte_Multiplexer : Byte_Multiplexers_Lib/Byte_Multiplexers_Lib/Byte_Multiplexer_4_to_1
  4_to_2_Encoder : Encoders_Lib/Encoders_Lib/Encoder_4_to_2
  Data_Out(1B) : Outport
  wires:
  From_Operand(1B)/1 -> 4_to_1_Byte_Multiplexer/4
  Reserved/1 -> 4_to_2_Encoder/1
  Select_Register(1b)/1 -> 4_to_2_Encoder/3
  From_Memory(1B)/1 -> 4_to_1_Byte_Multiplexer/6
  From_Register(1B)/1 -> 4_to_1_Byte_Multiplexer/5
  4_to_1_Byte_Multiplexer/1 -> Data_Out(1B)/1
  Select_Operand(1b)/1 -> 4_to_2_Encoder/2
  "Reserved "/1 -> 4_to_1_Byte_Multiplexer/3
  "Select_Memory(1b) "/1 -> 4_to_2_Encoder/4
  4_to_2_Encoder/2 -> 4_to_1_Byte_Multiplexer/2
  4_to_2_Encoder/1 -> 4_to_1_Byte_Multiplexer/1
